simulink model "eulerPropagate"  (R2023b)
settings: Solver=VariableStepAuto  StartTime=0.0  StopTime=Tfinal  MaxStep=3  RelTol=1e-3
values from neighbouring files (symbols this model uses):
  A_ptob = [0.00452111179393  0.994865050863  -0.101109297888; -0.99864921572  -0.000741813086313  -0.051953764597; -0.0517619888586  0.101207609816  0.993517848971]    [magConstants.mat]
  axesFlag = 0    [HW4main.m]    (also in plantConstants.m)
  I_sim = Itotal_p    [HW3main.m]    (also in HW4main.m; plantConstants.m = [17509.879164435788 0 0)
  Ir = 25    [HW4main.m]
  om0 = A_ptob' * [0 n_float 0].'    [HW4main.m]    (also in plantConstants.m = [-9.4694164366444919E-5; 0.00018515073030111903; 0.001829415)
  omr = omr + linPert.*rand(1)    [HW4main.m]
  r = A_ptob.' * [0 1 0].'    [HW4main.m]    (also in numerical_orbit_propagation.m = y(1:3); numerical_orbit_propagation_from_main.m = y(1:3))
settings Model: Creator=stanforduser  LastModifiedBy=kristopherriordan
settings DataIOCC: ExternalInput=[t,u]  SaveTime=off  ReturnWorkspaceOutputs=off  OutputSaveName=om

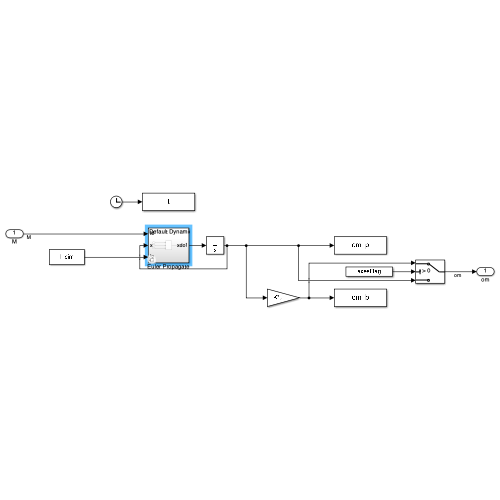
[thumbnail: Simulink's stored preview of the top-level diagram]
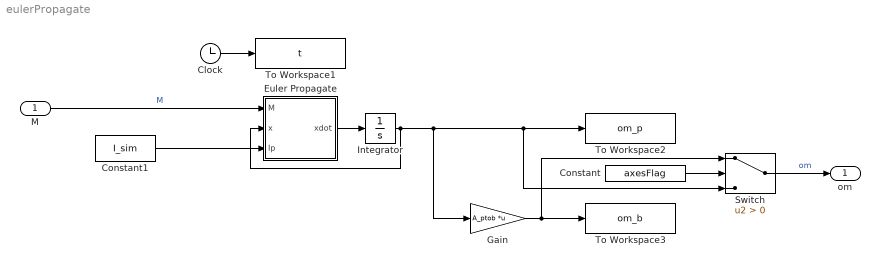
== system eulerPropagate ==
  M : Inport
  Clock : Clock
  Constant : Constant  Value=axesFlag
  Constant1 : Constant  Value=I_sim  VectorParams1D=off
  Euler Propagate : Subsystem  Variant=on  VariantControl=Euler Propagate
  Gain : Gain  Gain=A_ptob  Multiplication=Matrix(K*u)
  Integrator : Integrator  InitialCondition=om0
  Switch : Switch  Criteria=u2 > Threshold  SaturateOnIntegerOverflow=off  InputSameDT=off
  To Workspace1 : ToWorkspace  VariableName=t  SampleTime=-1
      settings: Save2DSignal=2-D array (concatenate along first dimension)
  To Workspace2 : ToWorkspace  VariableName=om_p  SampleTime=-1
      settings: Save2DSignal=2-D array (concatenate along first dimension)
  To Workspace3 : ToWorkspace  VariableName=om_b  SampleTime=-1
      settings: Save2DSignal=2-D array (concatenate along first dimension)
  om : Outport
  wires:
  Gain/1 -> To Workspace3/1, Switch/1
  Switch/1 -> om/1  "om"
  Integrator/1 -> To Workspace2/1, Switch/3, Gain/1, Euler Propagate/2(x)
  Constant/1 -> Switch/2
  Clock/1 -> To Workspace1/1
  M/1 -> Euler Propagate/1(M)  "M"
  Constant1/1 -> Euler Propagate/3(Ip)
  Euler Propagate/1(xdot) -> Integrator/1

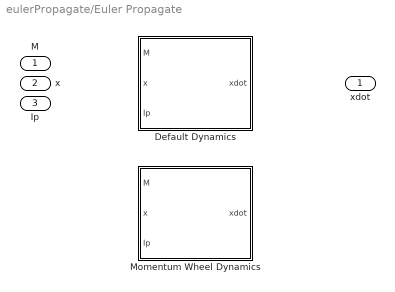
== system eulerPropagate/Euler Propagate ==
  M : Inport
  x : Inport  Port=2
  Ip : Inport  Port=3
  Default Dynamics : Subsystem  VariantControl="dynamicsType==\"default\""
  Momentum Wheel Dynamics : Subsystem  VariantControl="dynamicsType==\"wheel\""
  xdot : Outport

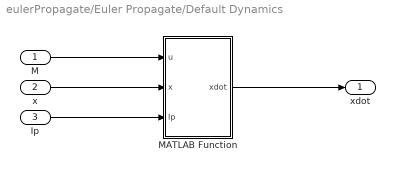
== system eulerPropagate/Euler Propagate/Default Dynamics ==
  M : Inport
  x : Inport  Port=2
  Ip : Inport  Port=3
  MATLAB Function : MATLAB Function  TreatAsAtomicUnit=on
  xdot : Outport
  wires:
  MATLAB Function/1(xdot) -> xdot/1
  Ip/1 -> MATLAB Function/3(Ip)
  M/1 -> MATLAB Function/1(u)
  x/1 -> MATLAB Function/2(x)

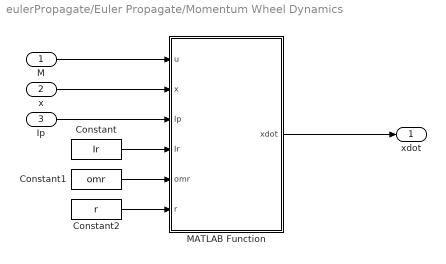
== system eulerPropagate/Euler Propagate/Momentum Wheel Dynamics ==
  M : Inport
  x : Inport  Port=2
  Ip : Inport  Port=3
  Constant : Constant  Value=Ir
  Constant1 : Constant  Value=omr
  Constant2 : Constant  Value=r  VectorParams1D=off
  MATLAB Function : MATLAB Function  TreatAsAtomicUnit=on
  xdot : Outport
  wires:
  MATLAB Function/1(xdot) -> xdot/1
  Ip/1 -> MATLAB Function/3(Ip)
  M/1 -> MATLAB Function/1(u)
  x/1 -> MATLAB Function/2(x)
  Constant/1 -> MATLAB Function/4(Ir)
  Constant1/1 -> MATLAB Function/5(omr)
  Constant2/1 -> MATLAB Function/6(r)

== matlab function eulerPropagate/Euler Propagate/Momentum Wheel Dynamics/MATLAB Function ==
  data: u input size=[3 1]; xdot output size=[3 1]; x input size=[3 1]; Ip input; Ir input; omr input; r input
function xdot = fcn(u,x,Ip,Ir,omr,r)

xdot = zeros(size(x));


Mx = u(1);
My = u(2);
Mz = u(3);

omx = x(1);
omy = x(2);
omz = x(3);

Ix = Ip(1,1);
Iy = Ip(2,2);
Iz = Ip(3,3);

rx = r(1);
ry = r(2);
rz = r(3);

wxdot = (1/Ix)*(Mx - (Iz - Iy)*omy*omz + Ir*omr*(omy*rz - omz*ry));
wydot = (1/Iy)*(My - (Ix - Iz)*omz*omx + Ir*omr*(omz*rx - omx*rz));
wzdot = (1/Iz)*(Mz - (Iy - Ix)*omx*omy + Ir*omr*(omx*ry - omy*rx));

xdot(1) = wxdot;
xdot(2) = wydot;
xdot(3) = wzdot;

end

== matlab function eulerPropagate/Euler Propagate/Default Dynamics/MATLAB Function ==
  data: u input size=[3 1]; xdot output size=[3 1]; x input size=[3 1]; Ip input
function xdot = fcn(u,x,Ip)

xdot = zeros(size(x));


Mx = u(1);
My = u(2);
Mz = u(3);

omx = x(1);
omy = x(2);
omz = x(3);

Ix = Ip(1,1);
Iy = Ip(2,2);
Iz = Ip(3,3);

wxdot = (1/Ix)*(Mx - (Iz - Iy)*omy*omz);
wydot = (1/Iy)*(My - (Ix - Iz)*omz*omx);
wzdot = (1/Iz)*(Mz - (Iy - Ix)*omx*omy);

xdot(1) = wxdot;
xdot(2) = wydot;
xdot(3) = wzdot;

end
